simulink model "torpedo_3"  (R2020a)
settings: Solver=VariableStepAuto  StartTime=0.0  StopTime=20  RelTol=1e-3
values from neighbouring files (symbols this model uses):
  k1 = 30    [torpedo.m]
  k2_1 = 1    [torpedo.m]
  k3 = 5    [torpedo.m]
  v = 10    [car_suspension.m]    (also in main.m = 20; torpedo.m = 40)
libraries: simulink x1
settings Model: Creator=ACER  LastModifiedBy=ACER

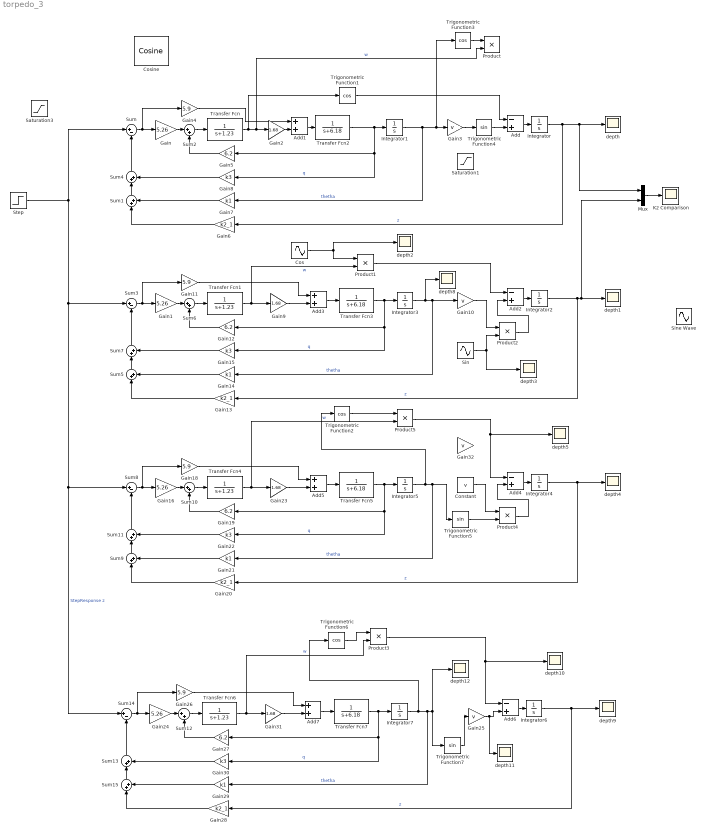
== system torpedo_3 ==
  Add{,2,4,6} (4 alike) : Sum  Inputs=-+
  Add{1,3,5,7} (4 alike) : Sum
  Constant : Constant  Value=v
  Cos : Sin  Phase=pi/2  Samples=2  SampleTime=0
  Cosine : simulink/Lookup Tables/Cosine  Formula=cos(2*pi*u)  NumDataPoints=(2^5)+1  OutputWordLength=16  InternalRulePriority=Speed
      settings: SourceProductBaseCode=SL
  Gain{,1,16,24} (4 alike) : Gain  Gain=5.26
  Gain{3,10,25,32} (4 alike) : Gain  Gain=v
  Gain{4,11,18,26} (4 alike) : Gain  Gain=5.9
  Gain{5,12,19,27} (4 alike) : Gain  Gain=6.2
  Gain{6,13,20,28} (4 alike) : Gain  Gain=k2_1
  Gain{7,14,21,29} (4 alike) : Gain  Gain=k1
  Gain{8,15,22,30} (4 alike) : Gain  Gain=k3
  Gain{2,9,23,31} (4 alike) : Gain  Gain=1.68
  Integrator{,1..7} (8 alike) : Integrator
  K2 Comparison : Scope
  Mux : Mux  Inputs=2
  Product{,1..5} (6 alike) : Product
  Saturation1 : Saturate  UpperLimit=5*(pi/180)  LowerLimit=-5*(pi/180)
  Saturation3 : Saturate  UpperLimit=5*(pi/180)  LowerLimit=-5*(pi/180)
  Sin : Sin  SampleTime=0
  Sine Wave : Sin  SampleTime=0
  Step : Step  SampleTime=0
  Sum{,3,8,14} (4 alike) : Sum  Inputs=|+-
  Sum{1..2,4..7,9..13,15} (12 alike) : Sum  Inputs=|++
  Transfer Fcn{,1,4,6} (4 alike) : TransferFcn  Denominator=[1 1.23]
  Transfer Fcn{2..3,5,7} (4 alike) : TransferFcn  Denominator=[1 6.18]
  Trigonometric Function{1..3,6} (4 alike) : Trigonometry  Operator=cos
  Trigonometric Function4 : Trigonometry
  Trigonometric Function5 : Trigonometry
  Trigonometric Function7 : Trigonometry
  depth{,1..5,8..12} (11 alike) : Scope
  wires:
  Sum3/1 -> Gain1/1, Gain11/1
  Gain11/1 -> Add3/1
  Gain12/1 -> Sum6/2
  Transfer Fcn3/1 -> Integrator3/1, Gain15/1, Gain12/1  "q"
  Gain1/1 -> Sum6/1
  Gain9/1 -> Add3/2
  Add2/1 -> Integrator2/1
  Gain15/1 -> Sum7/2
  Gain13/1 -> Sum5/1
  Gain14/1 -> Sum5/2
  Sum7/1 -> Sum3/2
  Integrator2/1 -> depth1/1, Mux/2, Gain13/1  "z"
  Integrator3/1 -> depth8/1, Gain10/1, Gain14/1  "thetha"
  Integrator1/1 -> Gain3/1, Trigonometric Function3/1, Gain7/1  "thetha"
  Sum5/1 -> Sum7/1
  Integrator/1 -> Mux/1, depth/1, Gain6/1  "z"
  Sum4/1 -> Sum/2
  Sum1/1 -> Sum4/1
  Gain8/1 -> Sum4/2
  Add3/1 -> Transfer Fcn3/1
  Gain6/1 -> Sum1/1
  Add/1 -> Integrator/1
  Gain2/1 -> Add1/2
  Transfer Fcn1/1 -> Product1/2, Gain9/1  "w"
  Transfer Fcn2/1 -> Integrator1/1, Gain8/1, Gain5/1  "q"
  Gain7/1 -> Sum1/2
  Gain/1 -> Sum2/1
  Gain4/1 -> Add1/1
  Gain5/1 -> Sum2/2
  Sum2/1 -> Transfer Fcn/1
  Mux/1 -> K2 Comparison/1
  Sum/1 -> Gain/1, Gain4/1
  Sum6/1 -> Transfer Fcn1/1
  Add1/1 -> Transfer Fcn2/1
  Transfer Fcn/1 -> Product/2, Gain2/1, Trigonometric Function1/1  "w"
  Gain3/1 -> Trigonometric Function4/1
  Trigonometric Function3/1 -> Product/1
  Trigonometric Function1/1 -> Add/1
  Trigonometric Function4/1 -> Add/2
  Cos/1 -> Product1/1, depth2/1
  Product1/1 -> Add2/1
  Gain10/1 -> Product2/1
  Sin/1 -> Product2/2, depth3/1
  Product2/1 -> Add2/2
  Product5/1 -> depth5/1, Add4/1
  Sum10/1 -> Transfer Fcn4/1
  Transfer Fcn4/1 -> Product5/2, Gain23/1  "w"
  Add5/1 -> Transfer Fcn5/1
  Sum9/1 -> Sum11/1
  Integrator5/1 -> Trigonometric Function2/1, Trigonometric Function5/1, Gain21/1  "thetha"
  Integrator4/1 -> depth4/1, Gain20/1  "z"
  Add4/1 -> Integrator4/1
  Sum11/1 -> Sum8/2
  Gain22/1 -> Sum11/2
  Gain20/1 -> Sum9/1
  Gain23/1 -> Add5/2
  Transfer Fcn5/1 -> Integrator5/1, Gain22/1, Gain19/1  "q"
  Gain16/1 -> Sum10/1
  Gain21/1 -> Sum9/2
  Gain18/1 -> Add5/1
  Gain19/1 -> Sum10/2
  Product4/1 -> Add4/2
  Constant/1 -> Product4/1
  Sum8/1 -> Gain16/1, Gain18/1
  Product3/1 -> depth10/1, Add6/1
  Gain26/1 -> Add7/1
  Gain27/1 -> Sum12/2
  Gain29/1 -> Sum15/2
  Gain24/1 -> Sum12/1
  Sum13/1 -> Sum14/2
  Add6/1 -> Integrator6/1
  Integrator6/1 -> depth9/1, Gain28/1  "z"
  Integrator7/1 -> Trigonometric Function6/1, depth12/1, Trigonometric Function7/1, Gain29/1  "thetha"
  Sum15/1 -> Sum13/1
  Transfer Fcn6/1 -> Product3/2, Gain31/1  "w"
  Add7/1 -> Transfer Fcn7/1
  Sum14/1 -> Gain24/1, Gain26/1
  Gain30/1 -> Sum13/2
  Sum12/1 -> Transfer Fcn6/1
  Step/1 -> Sum14/1, Sum8/1, Sum3/1, Sum/1  "StepResponse z"
  Trigonometric Function6/1 -> Product3/1
  Transfer Fcn7/1 -> Integrator7/1, Gain30/1, Gain27/1  "q"
  Gain28/1 -> Sum15/1
  Gain31/1 -> Add7/2
  Trigonometric Function7/1 -> Gain25/1
  Gain25/1 -> depth11/1, Add6/2
  Trigonometric Function2/1 -> Product5/1
  Trigonometric Function5/1 -> Product4/2
